simulink model "Model"  (R2018b)
settings: Solver=ode45  StartTime=0.0  StopTime=50  RelTol=1e-3  EnableMultiTasking=on
libraries: simulink x3, slident x1, re_lib x1
settings Model: Creator=Ultimate  LastModifiedBy=Mmd
settings DataIOCC: LimitDataPoints=on  SaveFormat=Array
settings OptimizationCC: LifeSpan=inf
settings DebuggingCC: UnderspecifiedInitializationDetection=Classic  MergeDetectMultiDrivingBlocksExec=none  SolverPrmCheckMsg=warning  StateNameClashWarn=warning  SFUnexpectedBacktrackingDiag=warning  SFNoUnconditionalDefaultTransitionDiag=warning  SFExecutionAtInitializationDiag=none
settings HardwareCC: ProdBitPerPointer=32  ProdBitPerSizeT=32  ProdBitPerPtrDiffT=32  ProdLargestAtomicFloat=None  ProdIntDivRoundTo=Undefined  ProdEndianess=Unspecified  ProdWordSize=32  ProdHWDeviceType=32-bit Generic
settings ModelReferenceCC: PropagateSignalLabelsOutOfModel=off
settings SFSimCC: SimUseLocalCustomCode=off
settings RTWCC: RTWUseLocalCustomCode=off
settings CodeAppCC: StateflowObjectComments=on
settings GRTTargetCC: TargetLangStandard=C89/C90 (ANSI)  GeneratePreprocessorConditionals=Disable all
settings ConfigComp: CovMetricSettings=dw  CovHtmlReporting=on  CovSaveCumulativeToWorkspaceVar=on  CovSaveSingleToWorkspaceVar=on  CovExternalEMLEnable=off  CovSFcnEnable=off

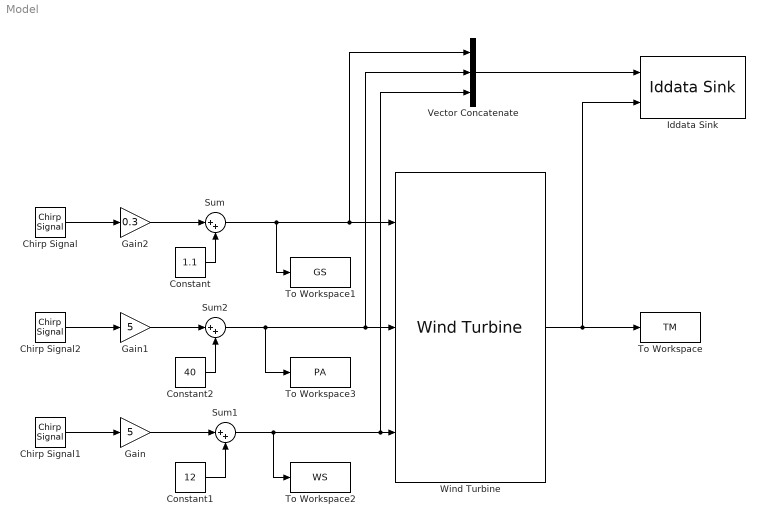
== system Model ==
  Chirp Signal : simulink/Sources/Chirp Signal  f1=0.1  T=40  f2=50
  Chirp Signal1 : simulink/Sources/Chirp Signal  f1=0.1  T=65  f2=50
  Chirp Signal2 : simulink/Sources/Chirp Signal  f1=0.1  T=75  f2=65
  Constant : Constant  Value=1.1
  Constant1 : Constant  Value=12
  Constant2 : Constant  Value=40
  Gain : Gain  Gain=5
  Gain1 : Gain  Gain=5
  Gain2 : Gain  Gain=0.3
  Iddata Sink : slident/Iddata Sink  datasetname=Data  Ts=0.1  isu=off  isy=off
      settings: SourceProductName=System Identification Toolbox  SourceProductBaseCode=ID
  Sum : Sum  Inputs=|++
  Sum1 : Sum  Inputs=|++
  Sum2 : Sum  Inputs=|++
  To Workspace : ToWorkspace  VariableName=TM  SampleTime=-1
  To Workspace1 : ToWorkspace  VariableName=GS  SampleTime=-1
  To Workspace2 : ToWorkspace  VariableName=WS  SampleTime=-1
  To Workspace3 : ToWorkspace  VariableName=PA  SampleTime=-1
  Vector Concatenate : Concatenate  NumInputs=3
  Wind Turbine : re_lib/Wind Generation/Wind Turbine  Pnom=1.5e6  Pelec_base=1.5e6/0.9  wind_base=12  P_wind_base=0.73  speed_nom=1.2  pitch_angle=0  c1_c6="[0.51763          116          0.4            5           21     0.006795]"  cp_nom=0.48  lambda_nom=8.1
      settings: SourceProductName=Simscape Electrical  SourceProductBaseCode=PS
  wires:
  Wind Turbine/1 -> To Workspace/1, Iddata Sink/2
  Constant/1 -> Sum/2
  Chirp Signal/1 -> Gain2/1
  Sum/1 -> Vector Concatenate/1, Wind Turbine/1, To Workspace1/1
  Constant1/1 -> Sum1/2
  Sum1/1 -> Vector Concatenate/3, Wind Turbine/3, To Workspace2/1
  Vector Concatenate/1 -> Iddata Sink/1
  Chirp Signal1/1 -> Gain/1
  Gain/1 -> Sum1/1
  Chirp Signal2/1 -> Gain1/1
  Gain1/1 -> Sum2/1
  Sum2/1 -> Vector Concatenate/2, Wind Turbine/2, To Workspace3/1
  Constant2/1 -> Sum2/2
  Gain2/1 -> Sum/1
